simulink model "crazyflie"  (R2019b)
settings: Solver=FixedStepDiscrete  StartTime=0.0  StopTime=160  FixedStep=0.01  RelTol=1e-3
values from neighbouring files (symbols this model uses):
  gamma = alpha / ( Ts + alpha )    (= 0.833333333333)    [lqr.m]
undefined symbols (not defined in the file or in its folder): DiscIntNeverNeededParam, Klqr
libraries: eeGeneralControl x4, simulink_extras x2
settings Model: PauseTimes=7  Creator=Zrean  LastModifiedBy=krthk
settings DataIOCC: ReturnWorkspaceOutputs=off
settings OptimizationCC: DefaultParameterBehavior=Inlined  UseDivisionForNetSlopeComputation=on  UseFloatMulNetSlope=on  UseSpecifiedMinMax=on  InlineInvariantSignals=on  PassReuseOutputArgsAs=Individual arguments  ZeroExternalMemoryAtStartup=off  ZeroInternalMemoryAtStartup=off  NoFixptDivByZeroProtection=on  EfficientFloat2IntCast=on  LifeSpan=1  EfficientTunableParamExpr=on
settings DebuggingCC: AlgebraicLoopMsg=error  ParameterTunabilityLossMsg=error  ArithmeticOperatorsInVariantConditions=warning
settings HardwareCC: ProdBitPerPointer=32  ProdBitPerSizeT=32  ProdBitPerPtrDiffT=32  ProdLargestAtomicInteger=Long  ProdLargestAtomicFloat=Double  ProdWordSize=32  ProdHWDeviceType=ARM Compatible->ARM Cortex
settings SFSimCC: SimUseLocalCustomCode=off  MATLABDynamicMemAlloc=off  CustomCodeUndefinedFunction=UseInterfaceOnly
settings RTWCC: SystemTargetFile=ert.tlc  GenCodeOnly=on  TemplateMakefile=ert_default_tmf  GenerateReport=on  RTWUseLocalCustomCode=off  BuildConfiguration=Faster Runs  IncludeHyperlinkInReport=on  LaunchReport=on  GenerateTraceInfo=on  GenerateTraceReport=on  GenerateTraceReportSl=on  GenerateTraceReportSf=on  GenerateTraceReportEml=on  GenerateCodeMetricsReport=on
settings CodeAppCC: ForceParamTrailComments=on  IgnoreCustomStorageClasses=off  OperatorAnnotations=on  SimulinkDataObjDesc=on  SFDataObjDesc=on  MATLABFcnDesc=on  InsertBlockDesc=on  StateflowObjectComments=on  MATLABSourceComments=on
settings ERTTargetCC: TargetLangStandard=C99 (ISO)  MultiwordLength=2048  CombineSignalStateStructs=on  SuppressErrorStatus=on  SupportAbsoluteTime=off  SupportNonFinite=off  SupportComplex=off  InlinedParameterPlacement=NonHierarchical  ERTCustomFileTemplate=crazyflie_wrapper.tlc  ERTFilePackagingFormat=CompactWithDataFile
settings SimscapeCC: SimscapeNormalizeSystem=off

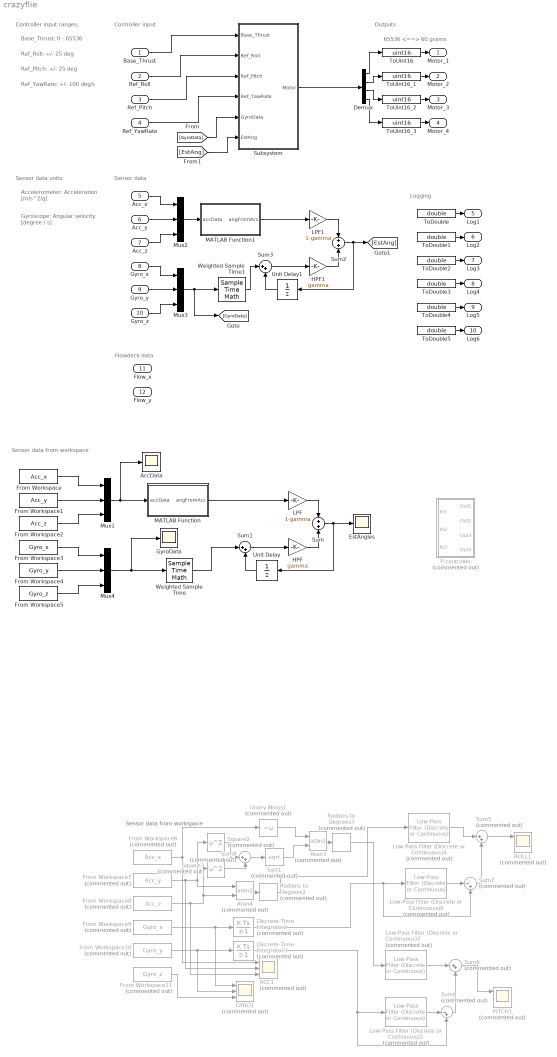
== system crazyflie ==
  note: 65536 <==> 60 grams
  note: Logging
  note: Outputs
  note: Sensor data
  note: Controller input
  note: Ref_Roll: +/- 25 deg
  note: Base_Thrust: 0 - 65536
  note: Ref_Pitch: +/- 25 deg
  note: Ref_YawRate: +/- 100 deg/s
  note: Controller input ranges:
  note: Gyroscope:
      | Angular velocity [degree / s]
  note: Accelerometer:
      | Acceleration [m/s^2/g]
  note: Sensor data units:
  note: Flowdeck data
  note: Sensor data from
      | workspace
  note: Sensor data from
      | workspace
  Base_Thrust : Inport  OutDataTypeStr=double
  Ref_Roll : Inport  Port=2  OutDataTypeStr=double
  Ref_Pitch : Inport  Port=3  OutDataTypeStr=double
  Ref_YawRate : Inport  Port=4  OutDataTypeStr=double
  Acc_x : Inport  Port=5  OutDataTypeStr=double  PortDimensions=1
  Acc_y : Inport  Port=6  OutDataTypeStr=double  PortDimensions=1
  Acc_z : Inport  Port=7  OutDataTypeStr=double  PortDimensions=1
  Gyro_x : Inport  Port=8  OutDataTypeStr=double  PortDimensions=1
  Gyro_y : Inport  Port=9  OutDataTypeStr=double  PortDimensions=1
  Gyro_z : Inport  Port=10  OutDataTypeStr=double  PortDimensions=1
  Flow_x : Inport  Port=11  OutDataTypeStr=int16  PortDimensions=1
  Flow_y : Inport  Port=12  OutDataTypeStr=int16  PortDimensions=1
  ACC1 : Scope  Commented=on  NumInputPorts=3
  AccData : Scope
  Atan3 : Trigonometry  Commented=on  Operator=atan2
  Atan4 : Trigonometry  Commented=on  Operator=atan2
  Demux : Demux
  Discrete-Time Integrator2 : DiscreteIntegrator  Commented=on  SampleTime=-1  ICPrevOutput=DiscIntNeverNeededParam  ICPrevScaledInput=DiscIntNeverNeededParam
  Discrete-Time Integrator3 : DiscreteIntegrator  Commented=on  SampleTime=-1  ICPrevOutput=DiscIntNeverNeededParam  ICPrevScaledInput=DiscIntNeverNeededParam
  EstAngles : Scope
  From Workspace : FromWorkspace  VariableName=Acc_x  OutDataTypeStr=double  SampleTime=0
  From Workspace1 : FromWorkspace  VariableName=Acc_y  OutDataTypeStr=double  SampleTime=0
  From Workspace10 : FromWorkspace  Commented=on  VariableName=Gyro_y  OutDataTypeStr=double  SampleTime=0
  From Workspace11 : FromWorkspace  Commented=on  VariableName=Gyro_z  OutDataTypeStr=double  SampleTime=0
  From Workspace2 : FromWorkspace  VariableName=Acc_z  OutDataTypeStr=double  SampleTime=0
  From Workspace3 : FromWorkspace  VariableName=Gyro_x  OutDataTypeStr=double  SampleTime=0
  From Workspace4 : FromWorkspace  VariableName=Gyro_y  OutDataTypeStr=double  SampleTime=0
  From Workspace5 : FromWorkspace  VariableName=Gyro_z  OutDataTypeStr=double  SampleTime=0
  From Workspace6 : FromWorkspace  Commented=on  VariableName=Acc_x  OutDataTypeStr=double  SampleTime=0
  From Workspace7 : FromWorkspace  Commented=on  VariableName=Acc_y  OutDataTypeStr=double  SampleTime=0
  From Workspace8 : FromWorkspace  Commented=on  VariableName=Acc_z  OutDataTypeStr=double  SampleTime=0
  From Workspace9 : FromWorkspace  Commented=on  VariableName=Gyro_x  OutDataTypeStr=double  SampleTime=0
  GYRO1 : Scope  Commented=on  NumInputPorts=3
  GyroData : Scope
  HPF : Gain  Gain=gamma
  HPF1 : Gain  Gain=gamma
  LPF : Gain  Gain=1-gamma
  LPF1 : Gain  Gain=1-gamma
  Low-Pass Filter (Discrete or Continuous){4..7} (4 alike) : eeGeneralControl/Low-Pass Filter (Discrete or Continuous)  Commented=on  K=1  T=1  B=inf  A=-inf  Ts=-1
      settings: SourceProductName=Simscape Electrical
  MATLAB Function : MATLAB Function  TreatAsAtomicUnit=on
  MATLAB Function1 : MATLAB Function  TreatAsAtomicUnit=on
  Mux{1..4} (4 alike) : Mux  Inputs=3
  P controller : Subsystem  Commented=on
  PITCH1 : Scope  Commented=on  NumInputPorts=3
  ROLL1 : Scope  Commented=on  NumInputPorts=3
  Radians to Degrees2 : simulink_extras/Transformations/Radians to Degrees  Commented=on
  Radians to Degrees3 : simulink_extras/Transformations/Radians to Degrees  Commented=on
  Sqrt1 : Sqrt  Commented=on  SaturateOnIntegerOverflow=on
  Square2 : Math  Commented=on  Operator=square  SignedPower=off  SaturateOnIntegerOverflow=on
  Square3 : Math  Commented=on  Operator=square  SignedPower=off  SaturateOnIntegerOverflow=on
  Subsystem : Subsystem
  Sum : Sum  Inputs=+|+
  Sum1 : Sum  Inputs=|++
  Sum2 : Sum  Inputs=+|+
  Sum3 : Sum  Inputs=|++
  Sum5 : Sum  Commented=on  Inputs=|++
  Sum6 : Sum  Commented=on  Inputs=|++
  Sum7 : Sum  Commented=on  Inputs=|-+
  Sum8 : Sum  Commented=on  Inputs=|-+
  Sum9 : Sum  Commented=on  Inputs=|++
  ToDouble{,1..5} (6 alike) : DataTypeConversion  OutDataTypeStr=double  SaturateOnIntegerOverflow=on
  ToUint16 : DataTypeConversion  OutDataTypeStr=uint16  SaturateOnIntegerOverflow=on
  ToUint16_1 : DataTypeConversion  OutDataTypeStr=uint16  SaturateOnIntegerOverflow=on
  ToUint16_2 : DataTypeConversion  OutDataTypeStr=uint16  SaturateOnIntegerOverflow=on
  ToUint16_3 : DataTypeConversion  OutDataTypeStr=uint16  SaturateOnIntegerOverflow=on
  Unary Minus1 : UnaryMinus  Commented=on
  Unit Delay : UnitDelay  SampleTime=-1  HasFrameUpgradeWarning=on
  Unit Delay1 : UnitDelay  SampleTime=-1  HasFrameUpgradeWarning=on
  Weighted Sample Time : SampleTimeMath  TsampMathOp=Ts Only
  Weighted Sample Time1 : SampleTimeMath  TsampMathOp=Ts Only
  Motor_1 : Outport  OutDataTypeStr=uint16  VectorParamsAs1DForOutWhenUnconnected=off  LockScale=on
  Motor_2 : Outport  Port=2  OutDataTypeStr=uint16  VectorParamsAs1DForOutWhenUnconnected=off  LockScale=on
  Motor_3 : Outport  Port=3  OutDataTypeStr=uint16  VectorParamsAs1DForOutWhenUnconnected=off  LockScale=on
  Motor_4 : Outport  Port=4  OutDataTypeStr=uint16  VectorParamsAs1DForOutWhenUnconnected=off  LockScale=on
  Log1 : Outport  Port=5  OutDataTypeStr=double  VectorParamsAs1DForOutWhenUnconnected=off
  Log2 : Outport  Port=6  OutDataTypeStr=double  VectorParamsAs1DForOutWhenUnconnected=off
  Log3 : Outport  Port=7  OutDataTypeStr=double  VectorParamsAs1DForOutWhenUnconnected=off
  Log4 : Outport  Port=8  OutDataTypeStr=double  VectorParamsAs1DForOutWhenUnconnected=off
  Log5 : Outport  Port=9  OutDataTypeStr=double  VectorParamsAs1DForOutWhenUnconnected=off
  Log6 : Outport  Port=10  OutDataTypeStr=double  VectorParamsAs1DForOutWhenUnconnected=off
  wires:
  ToUint16/1 -> Motor_1/1
  ToUint16_1/1 -> Motor_2/1
  ToUint16_2/1 -> Motor_3/1
  ToUint16_3/1 -> Motor_4/1
  ToDouble/1 -> Log1/1
  ToDouble1/1 -> Log2/1
  ToDouble2/1 -> Log3/1
  ToDouble3/1 -> Log4/1
  ToDouble4/1 -> Log5/1
  ToDouble5/1 -> Log6/1
  Sum5/1 -> ROLL1/1
  Low-Pass Filter (Discrete or Continuous)7/1 -> Sum6/1
  From Workspace11/1 -> GYRO1/3
  Atan3/1 -> Radians to Degrees3/1
  Discrete-Time Integrator2/1 -> Sum7/2, Low-Pass Filter (Discrete or Continuous)6/1
  Low-Pass Filter (Discrete or Continuous)6/1 -> Sum7/1
  Sum6/1 -> PITCH1/1
  Unary Minus1/1 -> Atan3/1
  Low-Pass Filter (Discrete or Continuous)5/1 -> Sum8/1
  Discrete-Time Integrator3/1 -> Sum8/2, Low-Pass Filter (Discrete or Continuous)5/1
  Sum8/1 -> Sum6/2
  Sum9/1 -> Sqrt1/1
  Radians to Degrees2/1 -> Low-Pass Filter (Discrete or Continuous)4/1
  Square3/1 -> Sum9/2
  From Workspace10/1 -> GYRO1/2, Discrete-Time Integrator3/1
  Sqrt1/1 -> Atan3/2
  Radians to Degrees3/1 -> Low-Pass Filter (Discrete or Continuous)7/1
  From Workspace8/1 -> ACC1/3, Square3/1, Atan4/2
  Sum7/1 -> Sum5/2
  From Workspace7/1 -> ACC1/2, Square2/1, Atan4/1
  From Workspace6/1 -> Unary Minus1/1, ACC1/1
  From Workspace9/1 -> GYRO1/1, Discrete-Time Integrator2/1
  Low-Pass Filter (Discrete or Continuous)4/1 -> Sum5/1
  Atan4/1 -> Radians to Degrees2/1
  Square2/1 -> Sum9/1
  From Workspace/1 -> Mux1/1
  From Workspace1/1 -> Mux1/2
  From Workspace2/1 -> Mux1/3
  From Workspace3/1 -> Mux4/1
  From Workspace4/1 -> Mux4/2
  From Workspace5/1 -> Mux4/3
  Mux1/1 -> AccData/1, MATLAB Function/1(accData)
  Mux4/1 -> GyroData/1, Weighted Sample Time/1
  LPF/1 -> Sum/1
  Sum1/1 -> HPF/1
  Weighted Sample Time/1 -> Sum1/1
  MATLAB Function/1(angFromAcc) -> LPF/1
  Unit Delay/1 -> Sum1/2
  HPF/1 -> Sum/2
  Sum/1 -> EstAngles/1, Unit Delay/1
  Demux/4 -> ToUint16_3/1
  Demux/2 -> ToUint16_1/1
  Demux/3 -> ToUint16_2/1
  Demux/1 -> ToUint16/1
  Subsystem/1(Motor) -> Demux/1
  Base_Thrust/1 -> Subsystem/1(Base_Thrust)
  Ref_Roll/1 -> Subsystem/2(Ref_Roll)
  Ref_Pitch/1 -> Subsystem/3(Ref_Pitch)
  Ref_YawRate/1 -> Subsystem/4(Ref_YawRate)
  [GyroData] -> Subsystem/5(GyroData)
  [EstAng] -> Subsystem/6(EstAng)
  Weighted Sample Time1/1 -> Sum3/1
  Acc_x/1 -> Mux2/1
  Gyro_x/1 -> Mux3/1
  Gyro_y/1 -> Mux3/2
  Acc_z/1 -> Mux2/3
  Gyro_z/1 -> Mux3/3
  MATLAB Function1/1(angFromAcc) -> LPF1/1
  Mux3/1 -> [GyroData], Weighted Sample Time1/1
  Acc_y/1 -> Mux2/2
  Sum2/1 -> Unit Delay1/1, [EstAng]
  LPF1/1 -> Sum2/1
  Sum3/1 -> HPF1/1
  Mux2/1 -> MATLAB Function1/1(accData)
  HPF1/1 -> Sum2/2
  Unit Delay1/1 -> Sum3/2

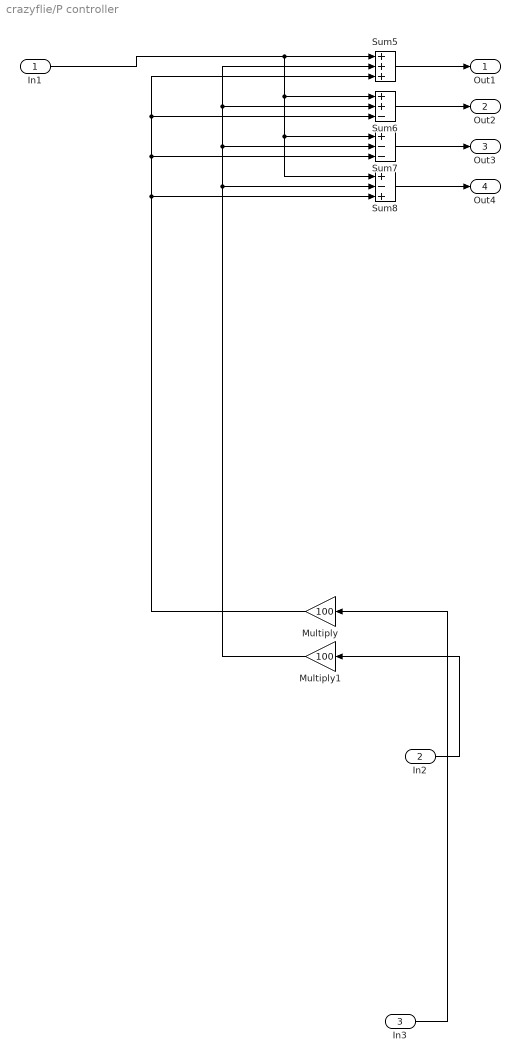
== system crazyflie/P controller ==
  In1 : Inport
  In2 : Inport  Port=2
  In3 : Inport  Port=3
  Multiply : Gain  Gain=100
  Multiply1 : Gain  Gain=100
  Sum5 : Sum  Inputs=+++
  Sum6 : Sum  Inputs=++-
  Sum7 : Sum  Inputs=+--
  Sum8 : Sum  Inputs=+-+
  Out1 : Outport
  Out2 : Outport  Port=2
  Out3 : Outport  Port=3
  Out4 : Outport  Port=4
  wires:
  Sum5/1 -> Out1/1
  In1/1 -> Sum7/1, Sum8/1, Sum6/1, Sum5/1
  Sum8/1 -> Out4/1
  In3/1 -> Multiply/1
  Multiply/1 -> Sum8/3, Sum7/3, Sum6/3, Sum5/3
  Multiply1/1 -> Sum8/2, Sum7/2, Sum6/2, Sum5/2
  Sum7/1 -> Out3/1
  Sum6/1 -> Out2/1
  In2/1 -> Multiply1/1

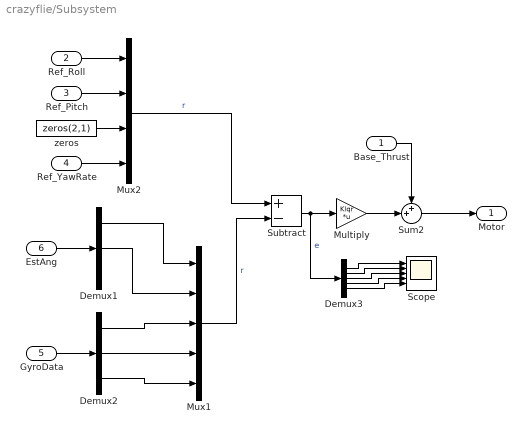
== system crazyflie/Subsystem ==
  Base_Thrust : Inport
  Ref_Roll : Inport  Port=2
  Ref_Pitch : Inport  Port=3
  Ref_YawRate : Inport  Port=4
  GyroData : Inport  Port=5
  EstAng : Inport  Port=6
  Demux1 : Demux  Outputs=3
  Demux2 : Demux  Outputs=3
  Demux3 : Demux  Outputs=5
  Multiply : Gain  Gain=Klqr  Multiplication=Matrix(K*u)
  Mux1 : Mux  Inputs=5
  Mux2 : Mux
  Scope : Scope  NumInputPorts=5
  Subtract : Sum  Inputs=+-
  Sum2 : Sum  Inputs=++|
  zeros : Constant  Value=zeros(2,1)
  Motor : Outport
  wires:
  Multiply/1 -> Sum2/2
  Base_Thrust/1 -> Sum2/1
  Sum2/1 -> Motor/1
  EstAng/1 -> Demux1/1
  Ref_Roll/1 -> Mux2/1
  Ref_Pitch/1 -> Mux2/2
  zeros/1 -> Mux2/3
  Ref_YawRate/1 -> Mux2/4
  Mux2/1 -> Subtract/1  "r"
  GyroData/1 -> Demux2/1
  Demux1/1 -> Mux1/1
  Demux1/2 -> Mux1/2
  Demux2/1 -> Mux1/3
  Demux2/2 -> Mux1/4
  Demux2/3 -> Mux1/5
  Mux1/1 -> Subtract/2  "r"
  Subtract/1 -> Demux3/1, Multiply/1  "e"
  Demux3/3 -> Scope/3
  Demux3/5 -> Scope/5
  Demux3/4 -> Scope/4
  Demux3/2 -> Scope/2
  Demux3/1 -> Scope/1

== matlab function crazyflie/MATLAB Function ==
  data: accData input; angFromAcc output
function angFromAcc = fcn(accData)

angFromAcc = [atan2(accData(2),accData(3)); 
    atan2(-accData(1),sqrt((accData(2))^2+(accData(3))^2)); 
    0];

== matlab function crazyflie/MATLAB Function1 ==
  data: accData input; angFromAcc output
function angFromAcc = fcn(accData)

angFromAcc = [atan2(accData(2),accData(3)); 
    atan2(-accData(1),sqrt((accData(2))^2+(accData(3))^2)); 
    0];
